simulink model "EspacioEstados_secador_solar"  (R2024b)
settings: Solver=VariableStepAuto  StartTime=0.0  StopTime=1000  RelTol=1e-3
values from neighbouring files (symbols this model uses):
  m_p_r = 0.02    [G.mat]
  T = 4.5    [tf2.mat]
  To_r = 58.83    [G.mat]
undefined symbols (not defined in the file or in its folder): C, G, H, K1, K2, Ke
settings Model: Creator=Celso  LastModifiedBy=syaba

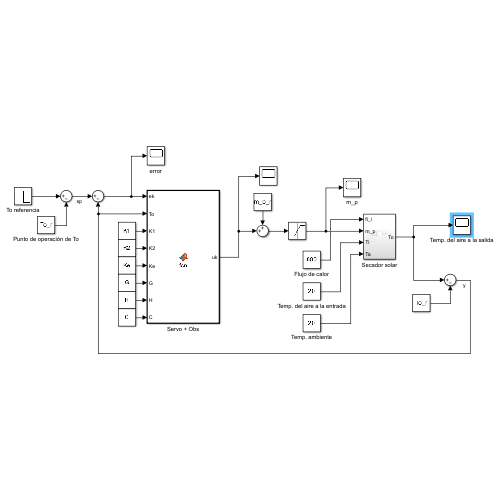
[thumbnail: Simulink's stored preview of the top-level diagram]
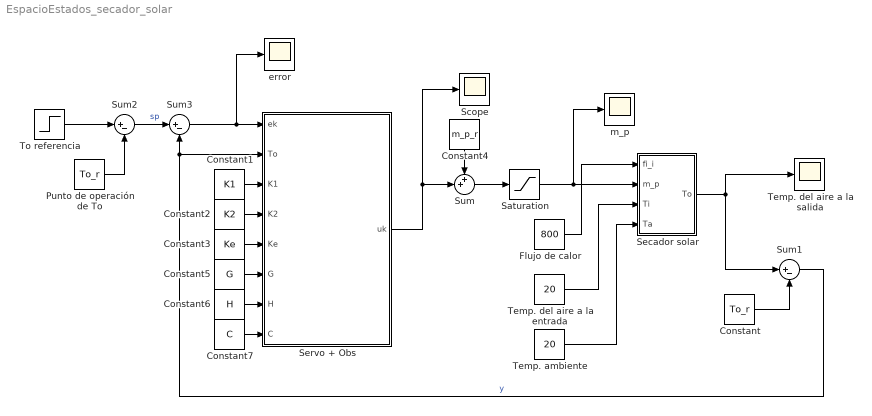
== system EspacioEstados_secador_solar ==
  Constant : Constant  Value=To_r
  Constant1 : Constant  Value=K1
  Constant2 : Constant  Value=K2  VectorParams1D=off
  Constant3 : Constant  Value=Ke  VectorParams1D=off
  Constant4 : Constant  Value=m_p_r
  Constant5 : Constant  Value=G  VectorParams1D=off
  Constant6 : Constant  Value=H  VectorParams1D=off
  Constant7 : Constant  Value=C  VectorParams1D=off
  Flujo de calor : Constant  Value=800
  Punto de operación de To : Constant  Value=To_r
  Saturation : Saturate  UpperLimit=0.1  LowerLimit=0
  Scope : Scope
  Secador solar : Subsystem
  Servo + Obs : MATLAB Function  TreatAsAtomicUnit=on  SystemSampleTime=T
  Sum : Sum  Inputs=++|
  Sum1 : Sum  Inputs=|+-
  Sum2 : Sum  Inputs=|+-
  Sum3 : Sum  Inputs=|+-
  Temp. ambiente : Constant  Value=20
  Temp. del aire a la entrada : Constant  Value=20
  Temp. del aire a la salida : Scope
  To referencia : Step  Time=500  Before=60  After=40  SampleTime=0
  error : Scope
  m_p : Scope
  wires:
  Temp. del aire a la entrada/1 -> Secador solar/3(Ti)
  Temp. ambiente/1 -> Secador solar/4(Ta)
  Secador solar/1(To) -> Sum1/1, Temp. del aire a la salida/1
  Flujo de calor/1 -> Secador solar/1(fi_i)
  Constant/1 -> Sum1/2
  To referencia/1 -> Sum2/1
  Punto de operación de To/1 -> Sum2/2
  Sum2/1 -> Sum3/1  "sp"
  Sum1/1 -> Sum3/2, Servo + Obs/2(To)  "y"
  Sum3/1 -> error/1, Servo + Obs/1(ek)
  Servo + Obs/1(uk) -> Scope/1, Sum/2
  Constant4/1 -> Sum/1
  Sum/1 -> Saturation/1
  Constant1/1 -> Servo + Obs/3(K1)
  Constant2/1 -> Servo + Obs/4(K2)
  Constant3/1 -> Servo + Obs/5(Ke)
  Constant5/1 -> Servo + Obs/6(G)
  Constant6/1 -> Servo + Obs/7(H)
  Constant7/1 -> Servo + Obs/8(C)
  Saturation/1 -> m_p/1, Secador solar/2(m_p)

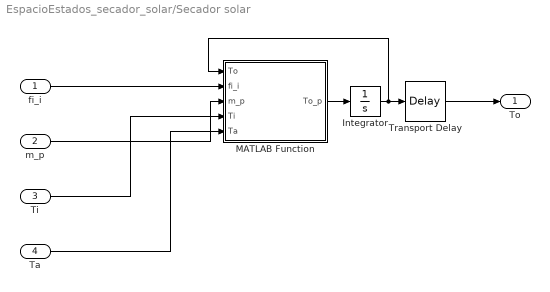
== system EspacioEstados_secador_solar/Secador solar ==
  fi_i : Inport
  m_p : Inport  Port=2
  Ti : Inport  Port=3
  Ta : Inport  Port=4
  Integrator : Integrator  InitialCondition=20
  MATLAB Function : MATLAB Function  TreatAsAtomicUnit=on
  Transport Delay : TransportDelay  DelayTime=10  InitialOutput=20
  To : Outport
  wires:
  Integrator/1 -> MATLAB Function/1(To), Transport Delay/1
  MATLAB Function/1(To_p) -> Integrator/1
  fi_i/1 -> MATLAB Function/2(fi_i)
  Ta/1 -> MATLAB Function/5(Ta)
  Ti/1 -> MATLAB Function/4(Ti)
  m_p/1 -> MATLAB Function/3(m_p)
  Transport Delay/1 -> To/1

== matlab function EspacioEstados_secador_solar/Servo + Obs ==
  data: ek input; To input; uk output; K1 input; K2 input; Ke input; G input; H input; C input
function uk = fcn(ek, To, K1, K2, Ke, G, H, C)

persistent vk_1;
persistent xob;

if isempty(vk_1)
    vk_1 = 0;
    xob = [0;0;0];
end;

vk = vk_1 + ek;
uk = K1*vk - K2*xob; 

%xob_m = xob(k+1)
% xob = xob(k)
xob_m = G*xob + H*uk + Ke*(To - C*xob);


vk_1 = vk;
xob = xob_m;

== matlab function EspacioEstados_secador_solar/Secador solar/MATLAB Function ==
  data: To input; To_p output; fi_i input; m_p input; Ti input; Ta input
function To_p = fcn(To,fi_i,m_p,Ti,Ta)

%Simula el calentamiento del aire en un secador solar
%To: temperatura del aire a la salida (°C)
%Ti: temperatura del aire a la entrada (°C)
%V: voltaje aplicado a la resistencia
%   eléctrica del calentador (volt)
%m_p: flujo de masa del aire que ingresa y sale del
%     secador solar (Kg/seg)
%Ta: temperatura ambiente (°C)

M = 0.9; %masa del aire en el secador solar (Kg)
c = 1005; %calor específico del aire (J/Kg-°C)
%fi_i = 800; %Flujo de calor proporcionada por la radiación solar
R = 2; %Resistencia térmica (°C.seg/J)


To_p = fi_i/(M*c) - m_p*(To-Ti)/M - (To-Ta)/(M*c*R)
